simulink model "model"  (R2019b)
settings: Solver=VariableStepAuto  StartTime=0.0  StopTime=sim_time  FixedStep=Ts/100  RelTol=1e-3
StopFcn:
  | %figure;plot(true_position.Data(:,1),true_position.Data(:,2))
  | 
  | figure;hold on;
  | plot(ref_pos.Data(:,1),ref_pos.Data(:,2));
  | plot(ref_pos_noLA.Data(:,1),ref_pos_noLA.Data(:,2));
  | plot(meas_pos.Data(:,1),meas_pos.Data(:,2));
  | title('Position');
  | xlabel('x (m)');
  | ylabel('y (m)');
  | legend('Reference Position','Reference Position without Look-Ahead','Measured Position');
values from neighbouring files (symbols this model uses):
  b = 1.095    [main.m]
  bike_params = [g h b a lambda m]    [main.m]
  complementary = 0.985    [main.m]
  D_balancing = 0.05    [main.m]
  D_heading = 0    [main.m]
  D_lateral = -0.0    (= 0)    [main.m]
  D_steering_position = 0    [main.m]
  g = 9.81    [main.m]
  g1_den = [1]    [main.m]
  g1_num = 3*[1]    [main.m]
  g2_den = [1]    [main.m]
  g2_num = 5*[1]    [main.m]
  heading_control = 1    [main.m]
  I_balancing = 0    [main.m]
  I_heading = 0    [main.m]
  I_lateral = -0.1    [main.m]
  I_steering_position = 30    [main.m]
  IMU_height = 0.45    [main.m]
  initial_roll = deg2rad(0)    [main.m]
  initial_rollrate = deg2rad(0)    [main.m]
  initial_x = 0    [main.m]
  initial_y = 0    [main.m]
  lambda = deg2rad(70)    [main.m]
  lateral_control = 1    [main.m]
  look_ahead = 0    [main.m]
  look_ahead_time = 2.0    (= 2)    [main.m]
  num_tf_steering = [253.4]    [main.m]
  P_balancing = 1    [main.m]
  P_heading = 0.1    [main.m]
  P_lateral = -0.1    [main.m]
  P_steering_position = 30    [main.m]
  path_tracking = 1    [main.m]
  path_x = path_x'    [paths.m]
  path_y = movmean(path_y,200)    [paths.m]
  roll_rate_coef = 0.9    [main.m]
  time_balance = 10    [main.m]
  Ts = 0.01    [main.m]
  v = 4    [main.m]
undefined symbols (not defined in the file or in its folder): A, B, C, cumulative_dist_along_path, curvature, D, den_filt_steeringrate, DiscIntNeverNeededParam, num_filt_steeringrate, Ts_IMU
libraries: simulink_extras x7, simulink x6, dspsigops x3, cstblocks x1
(part 1 of 2)
settings Model: Creator=maximef  LastModifiedBy=maximef
settings DataIOCC: ReturnWorkspaceOutputs=off
settings DebuggingCC: ArithmeticOperatorsInVariantConditions=warning
settings SFSimCC: CustomCodeUndefinedFunction=UseInterfaceOnly

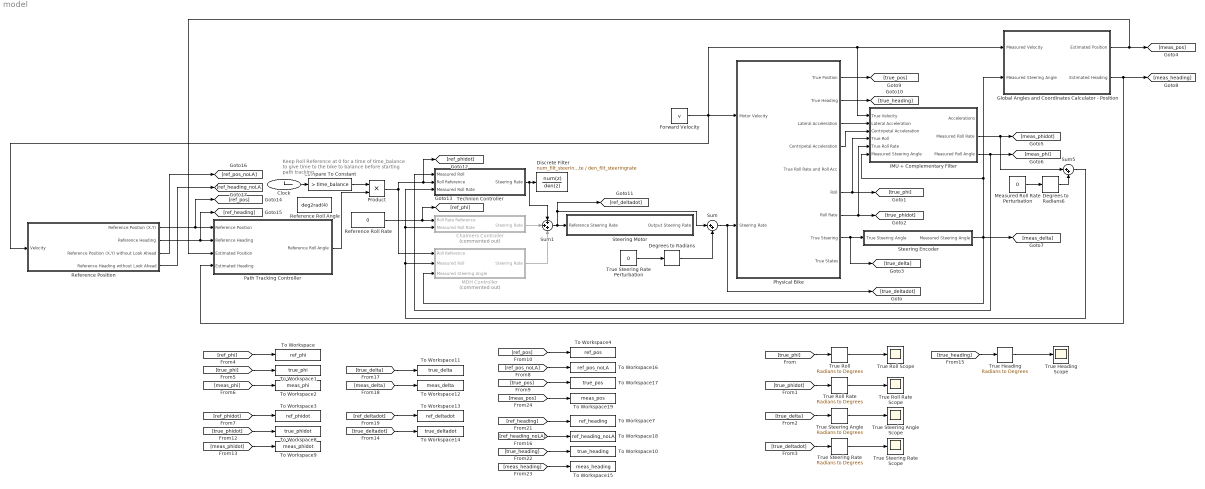
== system model ==
  note: Keep Roll Reference at 0 for a time of time_balance
      | to give time to the bike to balance before starting path tracking
  Chalmers Controller : Subsystem  Commented=on
  Clock : Clock
  Compare To Constant : simulink/Logic and Bit Operations/Compare To Constant  relop=>  const=time_balance  OutDataTypeStr=uint8
  Degrees to Radians : simulink_extras/Transformations/Degrees to Radians
  Degrees to Radians6 : simulink_extras/Transformations/Degrees to Radians
  Discrete Filter : DiscreteFilter  Numerator=num_filt_steeringrate  Denominator=den_filt_steeringrate  SampleTime=Ts
  Forward Velocity : Constant  Value=v
  Global Angles and Coordinates Calculator - Position : Subsystem  TreatAsAtomicUnit=on  SystemSampleTime=Ts
      settings: MinAlgLoopOccurrences=on
  IMU + Complementary Filter : Subsystem  TreatAsAtomicUnit=on
      settings: MinAlgLoopOccurrences=on
  MDH Controller : Subsystem  Commented=on
  Measured Roll Rate Perturbation : Constant  Value=0
  "Path Tracking Controller " : Subsystem  TreatAsAtomicUnit=on
      settings: MinAlgLoopOccurrences=on
  Physical Bike : Subsystem  TreatAsAtomicUnit=on
      settings: MinAlgLoopOccurrences=on
  Product : Product
  Reference Position : Subsystem  TreatAsAtomicUnit=on
      settings: MinAlgLoopOccurrences=on
  Reference Roll Angle : Constant  Value=deg2rad(4)
  Reference Roll Rate : Constant  Value=0
  Steering Encoder : Subsystem  TreatAsAtomicUnit=on  SystemSampleTime=Ts
  Steering Motor : Subsystem  TreatAsAtomicUnit=on
      settings: MinAlgLoopOccurrences=on
  Sum : Sum  Inputs=|++
  Sum1 : Sum  Inputs=+++
  Sum5 : Sum  Inputs=|++
  Technion Controller : Subsystem  TreatAsAtomicUnit=on
      settings: MinAlgLoopOccurrences=on
  To Workspace : ToWorkspace  VariableName=ref_phi  SaveFormat=Timeseries  SampleTime=-1
  To Workspace1 : ToWorkspace  VariableName=true_phi  SaveFormat=Timeseries  SampleTime=-1
  To Workspace10 : ToWorkspace  VariableName=true_heading  SaveFormat=Timeseries  SampleTime=-1
  To Workspace11 : ToWorkspace  VariableName=true_delta  SaveFormat=Timeseries  SampleTime=-1
  To Workspace12 : ToWorkspace  VariableName=meas_delta  SaveFormat=Timeseries  SampleTime=-1
  To Workspace13 : ToWorkspace  VariableName=ref_deltadot  SaveFormat=Timeseries  SampleTime=-1
  To Workspace14 : ToWorkspace  VariableName=true_deltadot  SaveFormat=Timeseries  SampleTime=-1
  To Workspace15 : ToWorkspace  VariableName=meas_heading  SaveFormat=Timeseries  SampleTime=-1
  To Workspace16 : ToWorkspace  VariableName=ref_pos_noLA  SaveFormat=Timeseries  SampleTime=-1
  To Workspace17 : ToWorkspace  VariableName=true_pos  SaveFormat=Timeseries  SampleTime=-1
  To Workspace18 : ToWorkspace  VariableName=ref_heading_noLA  SaveFormat=Timeseries  SampleTime=-1
  To Workspace19 : ToWorkspace  VariableName=meas_pos  SaveFormat=Timeseries  SampleTime=-1
  To Workspace2 : ToWorkspace  VariableName=meas_phi  SaveFormat=Timeseries  SampleTime=-1
  To Workspace3 : ToWorkspace  VariableName=ref_phidot  SaveFormat=Timeseries  SampleTime=-1
  To Workspace4 : ToWorkspace  VariableName=ref_pos  SaveFormat=Timeseries  SampleTime=-1
  To Workspace7 : ToWorkspace  VariableName=ref_heading  SaveFormat=Timeseries  SampleTime=-1
  To Workspace8 : ToWorkspace  VariableName=true_phidot  SaveFormat=Timeseries  SampleTime=-1
  To Workspace9 : ToWorkspace  VariableName=meas_phidot  SaveFormat=Timeseries  SampleTime=-1
  True Heading : simulink_extras/Transformations/Radians to Degrees
  True Heading Scope : Scope
  True Roll : simulink_extras/Transformations/Radians to Degrees
  True Roll Rate : simulink_extras/Transformations/Radians to Degrees
  True Roll Rate Scope : Scope
  True Roll Scope : Scope
  True Steering Angle : simulink_extras/Transformations/Radians to Degrees
  True Steering Angle Scope : Scope
  True Steering Rate : simulink_extras/Transformations/Radians to Degrees
  True Steering Rate Perturbation : Constant  Value=0
  True Steering Rate Scope : Scope
  wires:
  Measured Roll Rate Perturbation/1 -> Degrees to Radians6/1
  Physical Bike/6(Roll) -> [true_phi], IMU + Complementary Filter/4(True Roll)
  Sum/1 -> [true_deltadot], Physical Bike/2(Steering Rate)
  True Steering Rate Perturbation/1 -> Degrees to Radians/1
  Degrees to Radians/1 -> Sum/2
  Degrees to Radians6/1 -> Sum5/2
  Physical Bike/8(True Steering) -> [true_delta], Steering Encoder/1(True Steering Angle)
  Physical Bike/7(Roll Rate) -> [true_phidot], IMU + Complementary Filter/5(True Roll Rate)
  Sum5/1 -> MDH Controller/2(Measured Roll), Chalmers Controller/2(Measured Roll Rate), Technion Controller/3(Measured Roll Rate)
  Sum1/1 -> [ref_deltadot], Sum/1, Steering Motor/1(Reference Steering Rate)
  Steering Encoder/1(Measured Steering Angle) -> [meas_delta], MDH Controller/3(Measured Steering Angle), Global Angles and Coordinates Calculator - Position/2(Measured Steering Angle), IMU + Complementary Filter/6(Measured Steering Angle)
  Reference Position/2(Reference Heading) -> "Path Tracking Controller "/2(Reference Heading), [ref_heading]
  Forward Velocity/1 -> Reference Position/1(Velocity), IMU + Complementary Filter/1(True Velocity), Global Angles and Coordinates Calculator - Position/1(Measured Velocity), Physical Bike/1(Motor Velocity)
  Reference Position/1(Reference Position (X,Y)) -> "Path Tracking Controller "/1(Reference Position), [ref_pos]
  Physical Bike/3(Lateral Acceleration) -> IMU + Complementary Filter/2(Lateral Acceleration)
  Physical Bike/4(Centripetal Acceleration) -> IMU + Complementary Filter/3(Centripetal Acceleration)
  Global Angles and Coordinates Calculator - Position/1(Estimated Position) -> "Path Tracking Controller "/3(Estimated Position), [meas_pos]
  Global Angles and Coordinates Calculator - Position/2(Estimated Heading) -> "Path Tracking Controller "/4(Estimated Heading), [meas_heading]
  IMU + Complementary Filter/2(Measured Roll Rate) -> [meas_phidot], Sum5/1
  IMU + Complementary Filter/3(Measured Roll Angle) -> Technion Controller/1(Measured Roll), [meas_phi]
  Product/1 -> MDH Controller/1(Roll Reference), [ref_phidot], Technion Controller/2(Roll Reference)
  Reference Roll Rate/1 -> [ref_phi], Chalmers Controller/1(Roll Rate Reference)
  True Roll/1 -> True Roll Scope/1
  True Roll Rate/1 -> True Roll Rate Scope/1
  True Steering Angle/1 -> True Steering Angle Scope/1
  Physical Bike/1(True Position) -> [true_pos]
  Physical Bike/2(True Heading) -> [true_heading]
  [true_phi] -> True Roll/1
  [true_phidot] -> True Roll Rate/1
  [true_delta] -> True Steering Angle/1
  [true_deltadot] -> True Steering Rate/1
  True Steering Rate/1 -> True Steering Rate Scope/1
  [true_phi] -> To Workspace1/1
  [ref_phi] -> To Workspace/1
  [meas_phi] -> To Workspace2/1
  [ref_phidot] -> To Workspace3/1
  [meas_phidot] -> To Workspace9/1
  [true_phidot] -> To Workspace8/1
  [true_deltadot] -> To Workspace14/1
  [ref_deltadot] -> To Workspace13/1
  [meas_delta] -> To Workspace12/1
  [true_delta] -> To Workspace11/1
  [ref_heading] -> To Workspace7/1
  [ref_pos] -> To Workspace4/1
  [true_heading] -> True Heading/1
  True Heading/1 -> True Heading Scope/1
  Chalmers Controller/1(Steering Rate) -> Sum1/2
  MDH Controller/1(Steering Rate) -> Sum1/3
  Technion Controller/1(Steering Rate) -> Sum1/1, Discrete Filter/1
  Reference Position/3(Reference Position (X,Y) without Look Ahead) -> [ref_pos_noLA]
  Reference Position/4(Reference Heading without Look Ahead) -> [ref_heading_noLA]
  [meas_heading] -> To Workspace15/1
  [ref_heading_noLA] -> To Workspace18/1
  [true_heading] -> To Workspace10/1
  [true_pos] -> To Workspace17/1
  [ref_pos_noLA] -> To Workspace16/1
  [meas_pos] -> To Workspace19/1
  Clock/1 -> Compare To Constant/1
  "Path Tracking Controller "/1(Reference Roll Angle) -> Product/2
  Compare To Constant/1 -> Product/1

== system model/Chalmers Controller ==
  Roll Rate Reference : Inport
  Measured Roll Rate : Inport  Port=2
  Balance controller : simulink/Continuous/PID Controller  Controller=PID  Form=Parallel  TimeDomain=Discrete-time  SampleTime=Ts  IntegratorMethod=Forward Euler  FilterMethod=Forward Euler  ControllerParametersSource=internal  P=P_balancing  I=I_balancing  D=D_balancing  UseFilter=off  N=5  TunerSelectOption=Transfer Function Based (PID Tuner App)  InitialConditionSource=internal  InitialConditionForIntegrator=0  InitialConditionForFilter=0  DifferentiatorICPrevScaledInput=0  ExternalReset=none  TrackingMode=off  Kt=1  LimitOutput=off  UpperSaturationLimit=inf  LowerSaturationLimit=-inf  LinearizeAsGain=on  AntiWindupMode=none  Kb=1  POutMin=[]  POutMax=[]  IOutMin=[]  IOutMax=[]  DOutMin=[]  DOutMax=[]  NOutMin=[]  NOutMax=[]  SumOutMin=[]  SumOutMax=[]  SaturationOutMin=[]  SaturationOutMax=[]  PParamMin=[]  PParamMax=[]  IParamMin=[]  IParamMax=[]  DParamMin=[]  DParamMax=[]  NParamMin=[]  NParamMax=[]  KbParamMin=[]  KbParamMax=[]  KtParamMin=[]  KtParamMax=[]  KbOutMin=[]  KbOutMax=[]  KtOutMin=[]  KtOutMax=[]  IntegratorOutMin=[]  IntegratorOutMax=[]  FilterOutMin=[]  FilterOutMax=[]  SumI1OutMin=[]  SumI1OutMax=[]  SumI2OutMin=[]  SumI2OutMax=[]  SumI3OutMin=[]  SumI3OutMax=[]  SumI4OutMin=[]  SumI4OutMax=[]  SumDOutMin=[]  SumDOutMax=[]  DifferentiatorOutMin=[]  DifferentiatorOutMax=[]  FilterDiffOutCoefMin=[]  FilterDiffOutCoefMax=[]  ReciprocalOutMin=[]  ReciprocalOutMax=[]  SumDenOutMin=[]  SumDenOutMax=[]  SumNumOutMin=[]  SumNumOutMax=[]  DivideOutMin=[]  DivideOutMax=[]  IntegratorContinuousStateAttributes=''  IntegratorStateMustResolveToSignalObject=off  IntegratorRTWStateStorageClass=Auto  FilterContinuousStateAttributes=''  FilterStateMustResolveToSignalObject=off  FilterRTWStateStorageClass=Auto  ParallelPVariant=InternalParameters  IdealPVariant=Disabled  IVariant=InternalParameters  DVariant=InternalParameters  IntegratorVariant=Discrete  SatVariant=Disabled  AWVariant=Passthrough  PCopyVariant=Disabled  TRVariant=Disabled  FdbkBlocksVariant=Forward  IdealPFdbkVariant=Disabled  SatFdbkVariant=Disabled  DerivativeFilterVariant=Differentiator  NVariant=Passthrough  NCopyVariant=Disabled_SignalSpec  FilterICVariant=InternalICsDifferentiator  IntegratorICVariant=InternalICs  ExternalResetVariant=Disabled  TRSumVariant=Passthrough  SumFdbkVariant=Disabled  SumVariant=Sum_PID
  Sum1 : Sum  Inputs=|+-
  Steering Rate : Outport
  wires:
  Sum1/1 -> Balance controller/1
  Balance controller/1 -> Steering Rate/1
  Measured Roll Rate/1 -> Sum1/2
  Roll Rate Reference/1 -> Sum1/1

== system model/Global Angles and Coordinates Calculator - Position ==
  Measured Velocity : Inport
  Measured Steering Angle : Inport  Port=2
  Gain1 : Gain  Gain=sin(lambda)
  Measured Bike Angles to Global Angles : Subsystem
  Measured Global Angles to Global Coordinates : Subsystem
  Sum : Sum  Inputs=++|
  Estimated Position : Outport  VectorParamsAs1DForOutWhenUnconnected=off
  Estimated Heading : Outport  Port=2  VectorParamsAs1DForOutWhenUnconnected=off
  wires:
  Measured Bike Angles to Global Angles/1(Psi) -> Sum/2, Measured Global Angles to Global Coordinates/2(Psi)
  Gain1/1 -> Measured Bike Angles to Global Angles/2(Measured Steering Angle)
  Sum/1 -> Estimated Heading/1
  Measured Bike Angles to Global Angles/2(Beta) -> Sum/1, Measured Global Angles to Global Coordinates/3(Beta)
  Measured Global Angles to Global Coordinates/1("Position (X, Y)") -> Estimated Position/1
  Measured Velocity/1 -> Measured Global Angles to Global Coordinates/1(Velocity), Measured Bike Angles to Global Angles/1(Velocity)
  Measured Steering Angle/1 -> Gain1/1

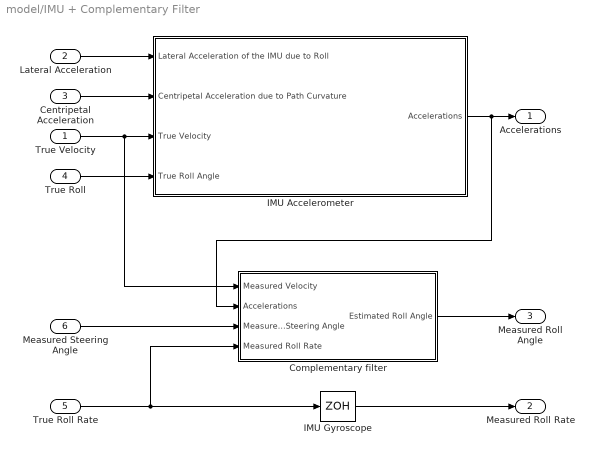
== system model/IMU + Complementary Filter ==
  True Velocity : Inport
  Lateral Acceleration : Inport  Port=2
  Centripetal Acceleration : Inport  Port=3
  True Roll : Inport  Port=4
  True Roll Rate : Inport  Port=5
  Measured Steering Angle : Inport  Port=6
  Complementary filter : Subsystem  SystemSampleTime=Ts_IMU
  IMU Accelerometer : Subsystem
  IMU Gyroscope : ZeroOrderHold  SampleTime=-1
  Accelerations : Outport  VectorParamsAs1DForOutWhenUnconnected=off
  Measured Roll Rate : Outport  Port=2  VectorParamsAs1DForOutWhenUnconnected=off
  Measured Roll Angle : Outport  Port=3  VectorParamsAs1DForOutWhenUnconnected=off
  wires:
  True Velocity/1 -> Complementary filter/1(Measured Velocity), IMU Accelerometer/3(True Velocity)
  Lateral Acceleration/1 -> IMU Accelerometer/1(Lateral Acceleration of the IMU due to Roll)
  Centripetal Acceleration/1 -> IMU Accelerometer/2(Centripetal Acceleration due to Path Curvature)
  True Roll/1 -> IMU Accelerometer/4(True Roll Angle)
  IMU Accelerometer/1(Accelerations) -> Complementary filter/2(Accelerations), Accelerations/1
  IMU Gyroscope/1 -> Measured Roll Rate/1
  True Roll Rate/1 -> Complementary filter/4(Measured Roll Rate), IMU Gyroscope/1
  Complementary filter/1(Estimated Roll Angle) -> Measured Roll Angle/1
  Measured Steering Angle/1 -> Complementary filter/3(Measured Steering Angle)

== system model/MDH Controller ==
  Roll Reference : Inport
  Measured Roll : Inport  Port=2
  Measured Steering Angle : Inport  Port=3
  Balance controller : simulink/Continuous/PID Controller  Controller=PID  Form=Parallel  TimeDomain=Discrete-time  SampleTime=Ts  IntegratorMethod=Forward Euler  FilterMethod=Forward Euler  ControllerParametersSource=internal  P=P_balancing  I=I_balancing  D=D_balancing  UseFilter=off  N=5  TunerSelectOption=Transfer Function Based (PID Tuner App)  InitialConditionSource=internal  InitialConditionForIntegrator=0  InitialConditionForFilter=0  DifferentiatorICPrevScaledInput=0  ExternalReset=none  TrackingMode=off  Kt=1  LimitOutput=off  UpperSaturationLimit=inf  LowerSaturationLimit=-inf  LinearizeAsGain=on  AntiWindupMode=none  Kb=1  POutMin=[]  POutMax=[]  IOutMin=[]  IOutMax=[]  DOutMin=[]  DOutMax=[]  NOutMin=[]  NOutMax=[]  SumOutMin=[]  SumOutMax=[]  SaturationOutMin=[]  SaturationOutMax=[]  PParamMin=[]  PParamMax=[]  IParamMin=[]  IParamMax=[]  DParamMin=[]  DParamMax=[]  NParamMin=[]  NParamMax=[]  KbParamMin=[]  KbParamMax=[]  KtParamMin=[]  KtParamMax=[]  KbOutMin=[]  KbOutMax=[]  KtOutMin=[]  KtOutMax=[]  IntegratorOutMin=[]  IntegratorOutMax=[]  FilterOutMin=[]  FilterOutMax=[]  SumI1OutMin=[]  SumI1OutMax=[]  SumI2OutMin=[]  SumI2OutMax=[]  SumI3OutMin=[]  SumI3OutMax=[]  SumI4OutMin=[]  SumI4OutMax=[]  SumDOutMin=[]  SumDOutMax=[]  DifferentiatorOutMin=[]  DifferentiatorOutMax=[]  FilterDiffOutCoefMin=[]  FilterDiffOutCoefMax=[]  ReciprocalOutMin=[]  ReciprocalOutMax=[]  SumDenOutMin=[]  SumDenOutMax=[]  SumNumOutMin=[]  SumNumOutMax=[]  DivideOutMin=[]  DivideOutMax=[]  IntegratorContinuousStateAttributes=''  IntegratorStateMustResolveToSignalObject=off  IntegratorRTWStateStorageClass=Auto  FilterContinuousStateAttributes=''  FilterStateMustResolveToSignalObject=off  FilterRTWStateStorageClass=Auto  ParallelPVariant=InternalParameters  IdealPVariant=Disabled  IVariant=InternalParameters  DVariant=InternalParameters  IntegratorVariant=Discrete  SatVariant=Disabled  AWVariant=Passthrough  PCopyVariant=Disabled  TRVariant=Disabled  FdbkBlocksVariant=Forward  IdealPFdbkVariant=Disabled  SatFdbkVariant=Disabled  DerivativeFilterVariant=Differentiator  NVariant=Passthrough  NCopyVariant=Disabled_SignalSpec  FilterICVariant=InternalICsDifferentiator  IntegratorICVariant=InternalICs  ExternalResetVariant=Disabled  TRSumVariant=Passthrough  SumFdbkVariant=Disabled  SumVariant=Sum_PID
  Steering Controller : simulink/Continuous/PID Controller  Controller=PID  Form=Parallel  TimeDomain=Discrete-time  SampleTime=Ts  IntegratorMethod=Forward Euler  FilterMethod=Forward Euler  ControllerParametersSource=internal  P=P_steering_position  I=I_steering_position  D=D_steering_position  UseFilter=off  N=100  TunerSelectOption=Transfer Function Based (PID Tuner App)  InitialConditionSource=internal  InitialConditionForIntegrator=0  InitialConditionForFilter=0  DifferentiatorICPrevScaledInput=0  ExternalReset=none  TrackingMode=off  Kt=1  LimitOutput=off  UpperSaturationLimit=inf  LowerSaturationLimit=-inf  LinearizeAsGain=on  AntiWindupMode=none  Kb=1  POutMin=[]  POutMax=[]  IOutMin=[]  IOutMax=[]  DOutMin=[]  DOutMax=[]  NOutMin=[]  NOutMax=[]  SumOutMin=[]  SumOutMax=[]  SaturationOutMin=[]  SaturationOutMax=[]  PParamMin=[]  PParamMax=[]  IParamMin=[]  IParamMax=[]  DParamMin=[]  DParamMax=[]  NParamMin=[]  NParamMax=[]  KbParamMin=[]  KbParamMax=[]  KtParamMin=[]  KtParamMax=[]  KbOutMin=[]  KbOutMax=[]  KtOutMin=[]  KtOutMax=[]  IntegratorOutMin=[]  IntegratorOutMax=[]  FilterOutMin=[]  FilterOutMax=[]  SumI1OutMin=[]  SumI1OutMax=[]  SumI2OutMin=[]  SumI2OutMax=[]  SumI3OutMin=[]  SumI3OutMax=[]  SumI4OutMin=[]  SumI4OutMax=[]  SumDOutMin=[]  SumDOutMax=[]  DifferentiatorOutMin=[]  DifferentiatorOutMax=[]  FilterDiffOutCoefMin=[]  FilterDiffOutCoefMax=[]  ReciprocalOutMin=[]  ReciprocalOutMax=[]  SumDenOutMin=[]  SumDenOutMax=[]  SumNumOutMin=[]  SumNumOutMax=[]  DivideOutMin=[]  DivideOutMax=[]  IntegratorContinuousStateAttributes=''  IntegratorStateMustResolveToSignalObject=off  IntegratorRTWStateStorageClass=Auto  FilterContinuousStateAttributes=''  FilterStateMustResolveToSignalObject=off  FilterRTWStateStorageClass=Auto  ParallelPVariant=InternalParameters  IdealPVariant=Disabled  IVariant=InternalParameters  DVariant=InternalParameters  IntegratorVariant=Discrete  SatVariant=Disabled  AWVariant=Passthrough  PCopyVariant=Disabled  TRVariant=Disabled  FdbkBlocksVariant=Forward  IdealPFdbkVariant=Disabled  SatFdbkVariant=Disabled  DerivativeFilterVariant=Differentiator  NVariant=Passthrough  NCopyVariant=Disabled_SignalSpec  FilterICVariant=InternalICsDifferentiator  IntegratorICVariant=InternalICs  ExternalResetVariant=Disabled  TRSumVariant=Passthrough  SumFdbkVariant=Disabled  SumVariant=Sum_PID
  Sum1 : Sum  Inputs=|+-
  Sum2 : Sum  Inputs=|+-
  Steering Rate : Outport
  wires:
  Sum2/1 -> Steering Controller/1
  Balance controller/1 -> Sum2/1
  Steering Controller/1 -> Steering Rate/1
  Measured Steering Angle/1 -> Sum2/2
  Measured Roll/1 -> Sum1/2
  Sum1/1 -> Balance controller/1
  Roll Reference/1 -> Sum1/1

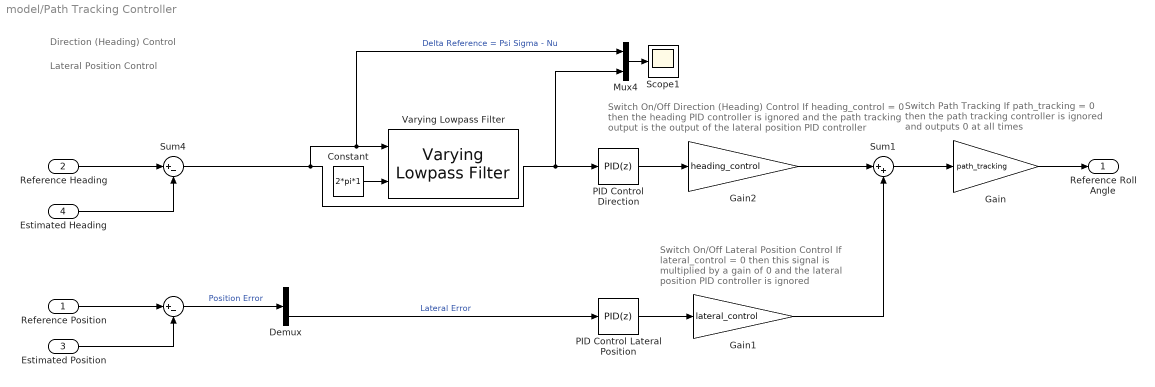
== system model/Path Tracking Controller  ==
  note: Direction (Heading) Control
  note: Lateral Position Control
  note: Switch On/Off Lateral Position Control
      | If lateral_control = 0 then this signal
      | is multiplied by a gain of 0 and the
      | lateral position PID controller is ignored
  note: Switch Path Tracking
      | If path_tracking = 0 then the path tracking controller
      | is ignored and outputs 0 at all times
  note: Switch On/Off Direction (Heading) Control
      | If heading_control = 0 then the heading PID controller is ignored
      | and the path tracking output is the output of the lateral position PID controller
  Reference Position : Inport
  Reference Heading : Inport  Port=2
  Estimated Position : Inport  Port=3
  Estimated Heading : Inport  Port=4
  " " : Sum  Inputs=|+-
  Constant : Constant  Value=2*pi*1
  Demux : Demux  Outputs=2
  Gain : Gain  Gain=path_tracking
  Gain1 : Gain  Gain=lateral_control
  Gain2 : Gain  Gain=heading_control
  Mux4 : Mux  Inputs=2
  PID Control Lateral Position : simulink/Continuous/PID Controller  Controller=PID  Form=Parallel  TimeDomain=Discrete-time  SampleTime=Ts  IntegratorMethod=Forward Euler  FilterMethod=Forward Euler  ControllerParametersSource=internal  P=P_lateral  I=I_lateral  D=D_lateral  UseFilter=on  N=100  TunerSelectOption=Transfer Function Based (PID Tuner App)  InitialConditionSource=internal  InitialConditionForIntegrator=0  InitialConditionForFilter=0  DifferentiatorICPrevScaledInput=0  ExternalReset=none  TrackingMode=off  Kt=1  LimitOutput=off  UpperSaturationLimit=inf  LowerSaturationLimit=-inf  LinearizeAsGain=on  AntiWindupMode=none  Kb=1  POutMin=[]  POutMax=[]  IOutMin=[]  IOutMax=[]  DOutMin=[]  DOutMax=[]  NOutMin=[]  NOutMax=[]  SumOutMin=[]  SumOutMax=[]  SaturationOutMin=[]  SaturationOutMax=[]  PParamMin=[]  PParamMax=[]  IParamMin=[]  IParamMax=[]  DParamMin=[]  DParamMax=[]  NParamMin=[]  NParamMax=[]  KbParamMin=[]  KbParamMax=[]  KtParamMin=[]  KtParamMax=[]  KbOutMin=[]  KbOutMax=[]  KtOutMin=[]  KtOutMax=[]  IntegratorOutMin=[]  IntegratorOutMax=[]  FilterOutMin=[]  FilterOutMax=[]  SumI1OutMin=[]  SumI1OutMax=[]  SumI2OutMin=[]  SumI2OutMax=[]  SumI3OutMin=[]  SumI3OutMax=[]  SumI4OutMin=[]  SumI4OutMax=[]  SumDOutMin=[]  SumDOutMax=[]  DifferentiatorOutMin=[]  DifferentiatorOutMax=[]  FilterDiffOutCoefMin=[]  FilterDiffOutCoefMax=[]  ReciprocalOutMin=[]  ReciprocalOutMax=[]  SumDenOutMin=[]  SumDenOutMax=[]  SumNumOutMin=[]  SumNumOutMax=[]  DivideOutMin=[]  DivideOutMax=[]  IntegratorContinuousStateAttributes=''  IntegratorStateMustResolveToSignalObject=off  IntegratorRTWStateStorageClass=Auto  FilterContinuousStateAttributes=''  FilterStateMustResolveToSignalObject=off  FilterRTWStateStorageClass=Auto  ParallelPVariant=InternalParameters  IdealPVariant=Disabled  IVariant=InternalParameters  DVariant=InternalParameters  IntegratorVariant=Discrete  SatVariant=Disabled  AWVariant=Passthrough  PCopyVariant=Disabled  TRVariant=Disabled  FdbkBlocksVariant=Forward  IdealPFdbkVariant=Disabled  SatFdbkVariant=Disabled  DerivativeFilterVariant=ForwardEulerFilter  NVariant=InternalParameters  NCopyVariant=Disabled  FilterICVariant=InternalICsFilter  IntegratorICVariant=InternalICs  ExternalResetVariant=Disabled  TRSumVariant=Passthrough  SumFdbkVariant=Disabled  SumVariant=Sum_PID
  PID Control Direction : simulink/Continuous/PID Controller  Controller=PID  Form=Parallel  TimeDomain=Discrete-time  SampleTime=Ts  IntegratorMethod=Forward Euler  FilterMethod=Forward Euler  ControllerParametersSource=internal  P=P_heading  I=I_heading  D=D_heading  UseFilter=off  N=100  TunerSelectOption=Transfer Function Based (PID Tuner App)  InitialConditionSource=internal  InitialConditionForIntegrator=0  InitialConditionForFilter=0  DifferentiatorICPrevScaledInput=0  ExternalReset=none  TrackingMode=off  Kt=1  LimitOutput=off  UpperSaturationLimit=inf  LowerSaturationLimit=-inf  LinearizeAsGain=on  AntiWindupMode=none  Kb=1  POutMin=[]  POutMax=[]  IOutMin=[]  IOutMax=[]  DOutMin=[]  DOutMax=[]  NOutMin=[]  NOutMax=[]  SumOutMin=[]  SumOutMax=[]  SaturationOutMin=[]  SaturationOutMax=[]  PParamMin=[]  PParamMax=[]  IParamMin=[]  IParamMax=[]  DParamMin=[]  DParamMax=[]  NParamMin=[]  NParamMax=[]  KbParamMin=[]  KbParamMax=[]  KtParamMin=[]  KtParamMax=[]  KbOutMin=[]  KbOutMax=[]  KtOutMin=[]  KtOutMax=[]  IntegratorOutMin=[]  IntegratorOutMax=[]  FilterOutMin=[]  FilterOutMax=[]  SumI1OutMin=[]  SumI1OutMax=[]  SumI2OutMin=[]  SumI2OutMax=[]  SumI3OutMin=[]  SumI3OutMax=[]  SumI4OutMin=[]  SumI4OutMax=[]  SumDOutMin=[]  SumDOutMax=[]  DifferentiatorOutMin=[]  DifferentiatorOutMax=[]  FilterDiffOutCoefMin=[]  FilterDiffOutCoefMax=[]  ReciprocalOutMin=[]  ReciprocalOutMax=[]  SumDenOutMin=[]  SumDenOutMax=[]  SumNumOutMin=[]  SumNumOutMax=[]  DivideOutMin=[]  DivideOutMax=[]  IntegratorContinuousStateAttributes=''  IntegratorStateMustResolveToSignalObject=off  IntegratorRTWStateStorageClass=Auto  FilterContinuousStateAttributes=''  FilterStateMustResolveToSignalObject=off  FilterRTWStateStorageClass=Auto  ParallelPVariant=InternalParameters  IdealPVariant=Disabled  IVariant=InternalParameters  DVariant=InternalParameters  IntegratorVariant=Discrete  SatVariant=Disabled  AWVariant=Passthrough  PCopyVariant=Disabled  TRVariant=Disabled  FdbkBlocksVariant=Forward  IdealPFdbkVariant=Disabled  SatFdbkVariant=Disabled  DerivativeFilterVariant=Differentiator  NVariant=Passthrough  NCopyVariant=Disabled_SignalSpec  FilterICVariant=InternalICsDifferentiator  IntegratorICVariant=InternalICs  ExternalResetVariant=Disabled  TRSumVariant=Passthrough  SumFdbkVariant=Disabled  SumVariant=Sum_PID
  Scope1 : Scope
  Sum1 : Sum  Inputs=|++
  Sum4 : Sum  Inputs=|+-
  Varying Lowpass Filter : cstblocks/Linear Parameter Varying/Varying Lowpass Filter  N=4
      settings: SourceProductName=Control System Toolbox
  Reference Roll Angle : Outport  VectorParamsAs1DForOutWhenUnconnected=off
  wires:
  Demux/2 -> PID Control Lateral Position/1  "Lateral Error"
  Estimated Position/1 -> " "/2
  " "/1 -> Demux/1  "Position Error"
  Sum4/1 -> Mux4/2, PID Control Direction/1, Mux4/1, Varying Lowpass Filter/1  "Delta Reference = Psi Sigma - Nu"
  Estimated Heading/1 -> Sum4/2
  PID Control Lateral Position/1 -> Gain1/1
  Reference Heading/1 -> Sum4/1
  Reference Position/1 -> " "/1
  Gain2/1 -> Sum1/1
  Sum1/1 -> Gain/1
  Gain/1 -> Reference Roll Angle/1
  PID Control Direction/1 -> Gain2/1
  Gain1/1 -> Sum1/2
  Mux4/1 -> Scope1/1
  Constant/1 -> Varying Lowpass Filter/2

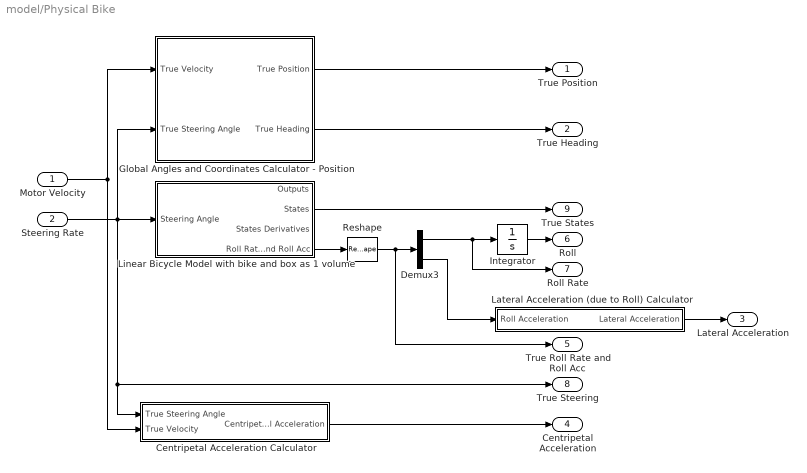
== system model/Physical Bike ==
  Motor Velocity : Inport
  Steering Rate : Inport  Port=2
  Centripetal Acceleration Calculator : Subsystem
  Demux3 : Demux  Outputs=2
  Global Angles and Coordinates Calculator - Position : Subsystem  SystemSampleTime=Ts
  Integrator : Integrator  InitialCondition=initial_roll
  Lateral Acceleration (due to Roll) Calculator : Subsystem
  Linear Bicycle Model with bike and box as 1 volume : Subsystem
  Reshape : Reshape
  True Position : Outport  VectorParamsAs1DForOutWhenUnconnected=off
  True Heading : Outport  Port=2  VectorParamsAs1DForOutWhenUnconnected=off
  Lateral Acceleration : Outport  Port=3  VectorParamsAs1DForOutWhenUnconnected=off
  Centripetal Acceleration : Outport  Port=4  VectorParamsAs1DForOutWhenUnconnected=off
  True Roll Rate and Roll Acc : Outport  Port=5  VectorParamsAs1DForOutWhenUnconnected=off
  Roll : Outport  Port=6  VectorParamsAs1DForOutWhenUnconnected=off
  Roll Rate : Outport  Port=7  VectorParamsAs1DForOutWhenUnconnected=off
  True Steering : Outport  Port=8  VectorParamsAs1DForOutWhenUnconnected=off
  True States : Outport  Port=9  VectorParamsAs1DForOutWhenUnconnected=off
  wires:
  Steering Rate/1 -> Linear Bicycle Model with bike and box as 1 volume/1(Steering Angle), Global Angles and Coordinates Calculator - Position/2(True Steering Angle), True Steering/1, Centripetal Acceleration Calculator/1(True Steering Angle)
  Centripetal Acceleration Calculator/1(Centripetal Acceleration) -> Centripetal Acceleration/1
  Demux3/2 -> Lateral Acceleration (due to Roll) Calculator/1(Roll Acceleration)
  Lateral Acceleration (due to Roll) Calculator/1(Lateral Acceleration) -> Lateral Acceleration/1
  Linear Bicycle Model with bike and box as 1 volume/2(States) -> True States/1
  Demux3/1 -> Integrator/1, Roll Rate/1
  Reshape/1 -> True Roll Rate and Roll Acc/1, Demux3/1
  Linear Bicycle Model with bike and box as 1 volume/4(Roll Rate and Roll Acc) -> Reshape/1
  Motor Velocity/1 -> Centripetal Acceleration Calculator/2(True Velocity), Global Angles and Coordinates Calculator - Position/1(True Velocity)
  Global Angles and Coordinates Calculator - Position/1(True Position) -> True Position/1
  Global Angles and Coordinates Calculator - Position/2(True Heading) -> True Heading/1
  Integrator/1 -> Roll/1

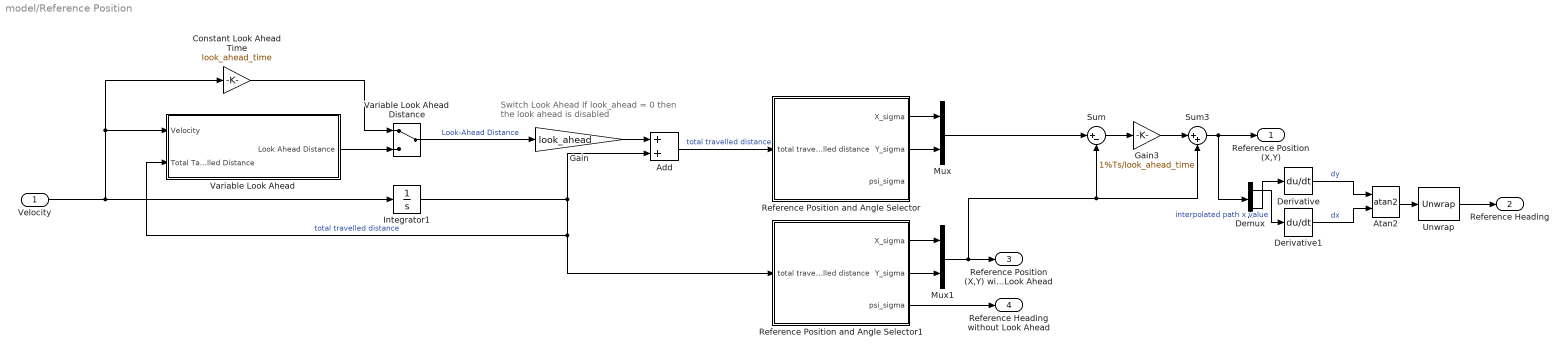
== system model/Reference Position ==
  note: Switch Look Ahead
      | If look_ahead = 0 then the look ahead is disabled
  Velocity : Inport
  Add : Sum
  Atan2 : Trigonometry  Operator=atan2
  Constant Look Ahead Time : Gain  Gain=look_ahead_time
  Demux : Demux  Outputs=2
  Derivative : Derivative
  Derivative1 : Derivative
  Gain : Gain  Gain=look_ahead
  Gain3 : Gain  Gain=1%Ts/look_ahead_time
  Integrator1 : Integrator
  Mux : Mux  Inputs=2
  Mux1 : Mux  Inputs=2
  Reference Position and Angle Selector : Subsystem
  Reference Position and Angle Selector1 : Subsystem
  Sum : Sum  Inputs=|+-
  Sum3 : Sum  Inputs=|++
  Unwrap : dspsigops/Unwrap  tol=pi  InputProcessing=Columns as channels (frame based)  running=off
  Variable Look Ahead Distance : ManualSwitch
  Variable Look Ahead : Subsystem
  Reference Position (X,Y) : Outport  VectorParamsAs1DForOutWhenUnconnected=off
  Reference Heading : Outport  Port=2  VectorParamsAs1DForOutWhenUnconnected=off
  Reference Position (X,Y) without Look Ahead : Outport  Port=3  VectorParamsAs1DForOutWhenUnconnected=off
  Reference Heading without Look Ahead : Outport  Port=4  VectorParamsAs1DForOutWhenUnconnected=off
  wires:
  Velocity/1 -> Integrator1/1, Constant Look Ahead Time/1, Variable Look Ahead/1(Velocity)
  Reference Position and Angle Selector/2(Y_sigma) -> Mux/2
  Add/1 -> Reference Position and Angle Selector/1(total travelled distance)  "total travelled distance"
  Reference Position and Angle Selector/1(X_sigma) -> Mux/1
  Variable Look Ahead Distance/1 -> Gain/1  "Look-Ahead Distance"
  Integrator1/1 -> Add/2, Reference Position and Angle Selector1/1(total travelled distance), Variable Look Ahead/2(Total Tavelled Distance)  "total travelled distance"
  Constant Look Ahead Time/1 -> Variable Look Ahead Distance/1
  Variable Look Ahead/1(Look Ahead Distance) -> Variable Look Ahead Distance/2
  Gain/1 -> Add/1
  Reference Position and Angle Selector1/2(Y_sigma) -> Mux1/2
  Reference Position and Angle Selector1/1(X_sigma) -> Mux1/1
  Mux1/1 -> Sum3/2, Sum/2, Reference Position (X,Y) without Look Ahead/1
  Reference Position and Angle Selector1/3(psi_sigma) -> Reference Heading without Look Ahead/1
  Gain3/1 -> Sum3/1
  Sum/1 -> Gain3/1
  Sum3/1 -> Demux/1, Reference Position (X,Y)/1
  Mux/1 -> Sum/1
  Atan2/1 -> Unwrap/1
  Demux/1 -> Derivative1/1  "interpolated path x value"
  Derivative1/1 -> Atan2/2  "dx"
  Derivative/1 -> Atan2/1  "dy"
  Unwrap/1 -> Reference Heading/1
  Demux/2 -> Derivative/1

== system model/Steering Encoder ==
  True Steering Angle : Inport
  Zero-Order Hold : ZeroOrderHold  SampleTime=Ts
  Measured Steering Angle : Outport  VectorParamsAs1DForOutWhenUnconnected=off
  wires:
  True Steering Angle/1 -> Zero-Order Hold/1
  Zero-Order Hold/1 -> Measured Steering Angle/1

== system model/Steering Motor ==
  Reference Steering Rate : Inport
  Steering motor transfer function Steering Rate reference to Steering Rate : TransferFcn  Numerator=[num_tf_steering]  Denominator=[den_tf_steering(1:end-1)]
  Output Steering Rate : Outport  VectorParamsAs1DForOutWhenUnconnected=off
  wires:
  Steering motor transfer function Steering Rate reference to Steering Rate/1 -> Output Steering Rate/1
  Reference Steering Rate/1 -> Steering motor transfer function Steering Rate reference to Steering Rate/1

== system model/Technion Controller ==
  Measured Roll : Inport
  Roll Reference : Inport  Port=2
  Measured Roll Rate : Inport  Port=3
  G1 : TransferFcn  Numerator=g1_num  Denominator=g1_den
  G2 : TransferFcn  Numerator=g2_num  Denominator=g2_den
  Sum4 : Sum  Inputs=|+-
  Sum6 : Sum  Inputs=|+-
  Steering Rate : Outport
  wires:
  G1/1 -> Sum4/1
  Sum4/1 -> G2/1
  Roll Reference/1 -> Sum6/1
  Sum6/1 -> G1/1
  Measured Roll/1 -> Sum6/2
  G2/1 -> Steering Rate/1
  Measured Roll Rate/1 -> Sum4/2

== system model/Global Angles and Coordinates Calculator - Position/Measured Bike Angles to Global Angles ==
  Velocity : Inport
  Measured Steering Angle : Inport  Port=2
  " Bike Parameters Model " : Constant  Value=bike_params
  Discrete-Time Integrator : DiscreteIntegrator  SampleTime=-1  ICPrevOutput=DiscIntNeverNeededParam  ICPrevScaledInput=DiscIntNeverNeededParam
  Integrator : Integrator  Commented=on
  MATLAB Function : MATLAB Function  TreatAsAtomicUnit=on
  Psi : Outport  VectorParamsAs1DForOutWhenUnconnected=off
  Beta : Outport  Port=2  VectorParamsAs1DForOutWhenUnconnected=off
  wires:
  MATLAB Function/2(beta) -> Beta/1
  MATLAB Function/1(psi_d) -> Discrete-Time Integrator/1
  Discrete-Time Integrator/1 -> Psi/1
  " Bike Parameters Model "/1 -> MATLAB Function/2(parameters_model)
  Measured Steering Angle/1 -> MATLAB Function/3(delta)
  Velocity/1 -> MATLAB Function/1(v)

== system model/Global Angles and Coordinates Calculator - Position/Measured Global Angles to Global Coordinates ==
  Velocity : Inport
  Psi : Inport  Port=2
  Beta : Inport  Port=3
  Discrete-Time Integrator : DiscreteIntegrator  InitialCondition=initial_x  SampleTime=-1  ICPrevOutput=DiscIntNeverNeededParam  ICPrevScaledInput=DiscIntNeverNeededParam
  Discrete-Time Integrator1 : DiscreteIntegrator  InitialCondition=initial_y  SampleTime=-1  ICPrevOutput=DiscIntNeverNeededParam  ICPrevScaledInput=DiscIntNeverNeededParam
  Integrator1 : Integrator  Commented=on  InitialCondition=initial_x
  Integrator2 : Integrator  Commented=on  InitialCondition=initial_y
  MATLAB Function1 : MATLAB Function  TreatAsAtomicUnit=on
  Mux : Mux  Inputs=2
  "Position (X, Y)" : Outport  VectorParamsAs1DForOutWhenUnconnected=off
  wires:
  MATLAB Function1/2(Ydot) -> Discrete-Time Integrator1/1  "Ydot"
  MATLAB Function1/1(Xdot) -> Discrete-Time Integrator/1  "Xdot"
  Psi/1 -> MATLAB Function1/2(psi)
  Beta/1 -> MATLAB Function1/3(beta)
  Velocity/1 -> MATLAB Function1/1(v)
  Discrete-Time Integrator1/1 -> Mux/2
  Discrete-Time Integrator/1 -> Mux/1
  Mux/1 -> "Position (X, Y)"/1

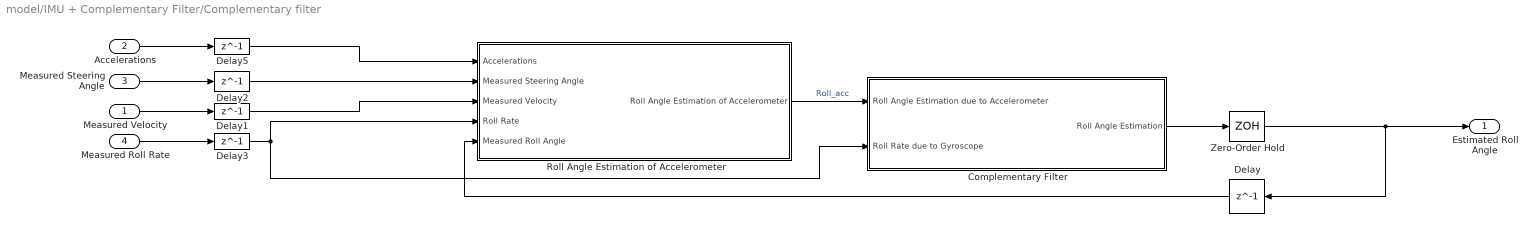
== system model/IMU + Complementary Filter/Complementary filter ==
  Measured Velocity : Inport
  Accelerations : Inport  Port=2
  Measured Steering Angle : Inport  Port=3
  Measured Roll Rate : Inport  Port=4
  Complementary Filter : Subsystem  TreatAsAtomicUnit=on  SystemSampleTime=Ts
  Delay{,1..3,5} (5 alike) : Delay  DelayLength=1
  Roll Angle Estimation of Accelerometer : Subsystem
  Zero-Order Hold : ZeroOrderHold  SampleTime=Ts
  Estimated Roll Angle : Outport  VectorParamsAs1DForOutWhenUnconnected=off
  wires:
  Roll Angle Estimation of Accelerometer/1(Roll Angle Estimation of Accelerometer) -> Complementary Filter/1(Roll Angle Estimation due to Accelerometer)  "Roll_acc"
  Measured Roll Rate/1 -> Delay3/1
  Accelerations/1 -> Delay5/1
  Measured Steering Angle/1 -> Delay2/1
  Measured Velocity/1 -> Delay1/1
  Delay/1 -> Roll Angle Estimation of Accelerometer/5(Measured Roll Angle)
  Delay1/1 -> Roll Angle Estimation of Accelerometer/3(Measured Velocity)
  Delay2/1 -> Roll Angle Estimation of Accelerometer/2(Measured Steering Angle)
  Delay3/1 -> Roll Angle Estimation of Accelerometer/4(Roll Rate), Complementary Filter/2(Roll Rate due to Gyroscope)
  Delay5/1 -> Roll Angle Estimation of Accelerometer/1(Accelerations)
  Complementary Filter/1(Roll Angle Estimation) -> Zero-Order Hold/1
  Zero-Order Hold/1 -> Estimated Roll Angle/1, Delay/1

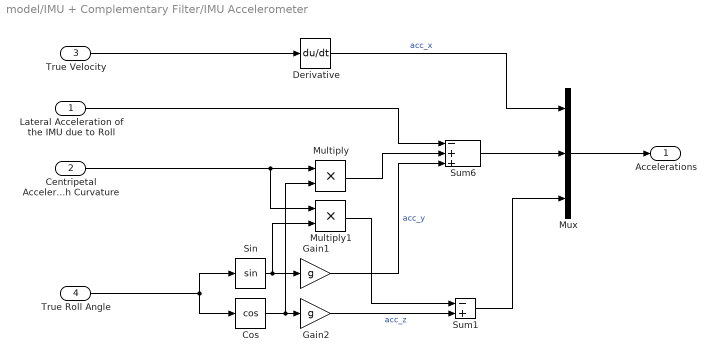
== system model/IMU + Complementary Filter/IMU Accelerometer ==
  Lateral Acceleration of the IMU due to Roll : Inport
  Centripetal Acceleration due to Path Curvature : Inport  Port=2
  True Velocity : Inport  Port=3
  True Roll Angle : Inport  Port=4
  Cos : Trigonometry  Operator=cos
  Derivative : Derivative  CoefficientInTFapproximation=-1
  Gain1 : Gain  Gain=g
  Gain2 : Gain  Gain=g
  Multiply : Product
  Multiply1 : Product
  Mux : Mux  Inputs=3
  Sin : Trigonometry
  Sum1 : Sum  Inputs=-+
  Sum6 : Sum  Inputs=-++
  Accelerations : Outport  VectorParamsAs1DForOutWhenUnconnected=off
  wires:
  Multiply/1 -> Sum6/2
  Gain1/1 -> Sum6/3  "acc_y"
  Sin/1 -> Multiply1/2, Gain1/1
  Derivative/1 -> Mux/1  "acc_x"
  Cos/1 -> Multiply/2, Gain2/1
  Gain2/1 -> Sum1/2  "acc_z"
  True Roll Angle/1 -> Sin/1, Cos/1
  True Velocity/1 -> Derivative/1
  Centripetal Acceleration due to Path Curvature/1 -> Multiply1/1, Multiply/1
  Multiply1/1 -> Sum1/1
  Sum1/1 -> Mux/3
  Mux/1 -> Accelerations/1
  Sum6/1 -> Mux/2
  Lateral Acceleration of the IMU due to Roll/1 -> Sum6/1

== system model/Physical Bike/Centripetal Acceleration Calculator ==
  True Steering Angle : Inport
  True Velocity : Inport  Port=2
  Divide : Product  Inputs=*/
  Gain : Gain  Gain=sin(lambda)
  Multiply : Product
  Square : Math  Operator=square  SaturateOnIntegerOverflow=on
  Tan : Trigonometry  Operator=tan
  b Real Bike : Constant  Value=b
  Centripetal Acceleration : Outport  VectorParamsAs1DForOutWhenUnconnected=off
  wires:
  True Velocity/1 -> Square/1
  Square/1 -> Divide/1
  b Real Bike/1 -> Divide/2
  True Steering Angle/1 -> Gain/1
  Divide/1 -> Multiply/1
  Tan/1 -> Multiply/2
  Multiply/1 -> Centripetal Acceleration/1
  Gain/1 -> Tan/1

== system model/Physical Bike/Global Angles and Coordinates Calculator - Position ==
  note: True Steering
      | Angle
  True Velocity : Inport
  True Steering Angle : Inport  Port=2
  Gain1 : Gain  Gain=sin(lambda)
  Measured Bike Angles to Global Angles : Subsystem
  Measured Global Angles to Global Coordinates : Subsystem
  Sum : Sum  Inputs=++|
  True Position : Outport  VectorParamsAs1DForOutWhenUnconnected=off
  True Heading : Outport  Port=2  VectorParamsAs1DForOutWhenUnconnected=off
  wires:
  Measured Bike Angles to Global Angles/1(Psi) -> Sum/2, Measured Global Angles to Global Coordinates/2(Psi)
  Gain1/1 -> Measured Bike Angles to Global Angles/2(Measured Steering Angle)
  Sum/1 -> True Heading/1
  Measured Bike Angles to Global Angles/2(Beta) -> Sum/1, Measured Global Angles to Global Coordinates/3(Beta)
  Measured Global Angles to Global Coordinates/1("Position (X, Y)") -> True Position/1
  True Velocity/1 -> Measured Global Angles to Global Coordinates/1(Velocity), Measured Bike Angles to Global Angles/1(Velocity)
  True Steering Angle/1 -> Gain1/1

== system model/Physical Bike/Lateral Acceleration (due to Roll) Calculator ==
  Roll Acceleration : Inport
  Constant3 : Constant  Value=IMU_height
  Multiply : Product
  Lateral Acceleration : Outport  VectorParamsAs1DForOutWhenUnconnected=off
  wires:
  Multiply/1 -> Lateral Acceleration/1
  Constant3/1 -> Multiply/1
  Roll Acceleration/1 -> Multiply/2

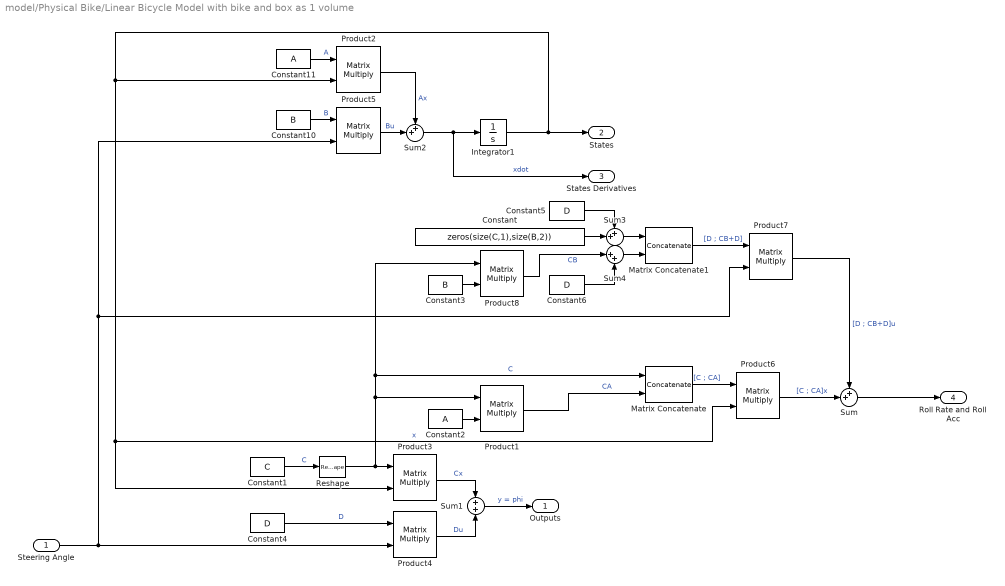
== system model/Physical Bike/Linear Bicycle Model with bike and box as 1 volume ==
  Steering Angle : Inport
  Constant : Constant  Value=zeros(size(C,1),size(B,2))
  Constant1 : Constant  Value=C
  Constant10 : Constant  Value=B
  Constant11 : Constant  Value=A
  Constant2 : Constant  Value=A
  Constant3 : Constant  Value=B
  Constant4 : Constant  Value=D
  Constant5 : Constant  Value=D
  Constant6 : Constant  Value=D
  Integrator1 : Integrator  InitialCondition=[C ; C*A]\[initial_rollrate ; 0]
  Matrix Concatenate : Concatenate  Mode=Multidimensional array
  Matrix Concatenate1 : Concatenate  Mode=Multidimensional array
  Product{1..8} (8 alike) : Product  SCDEnableBlockLinearizationSpecification=on  Multiplication=Matrix(*)
  Reshape : Reshape  OutputDimensionality=Customize  OutputDimensions=[size(C,1),size(C,2)]
  Sum : Sum  Inputs=++|
  Sum1 : Sum
  Sum2 : Sum  Inputs=++|
  Sum3 : Sum  Inputs=++|
  Sum4 : Sum  Inputs=|++
  Outputs : Outport  VectorParamsAs1DForOutWhenUnconnected=off
  States : Outport  Port=2  VectorParamsAs1DForOutWhenUnconnected=off
  States Derivatives : Outport  Port=3  VectorParamsAs1DForOutWhenUnconnected=off
  Roll Rate and Roll Acc : Outport  Port=4  VectorParamsAs1DForOutWhenUnconnected=off
  wires:
  Reshape/1 -> Product3/1, Product8/1, Matrix Concatenate/1, Product1/1  "C"
  Sum/1 -> Roll Rate and Roll Acc/1
  Constant1/1 -> Reshape/1  "C"
  Matrix Concatenate/1 -> Product6/1  "[C ; CA]"
  Product5/1 -> Sum2/2  "Bu"
  Matrix Concatenate1/1 -> Product7/1  "[D ; CB+D]"
  Constant11/1 -> Product2/1  "A"
  Constant3/1 -> Product8/2
  Product6/1 -> Sum/2  "[C ; CA]x"
  Sum2/1 -> Integrator1/1, States Derivatives/1  "xdot"
  Product2/1 -> Sum2/1  "Ax"
  Product1/1 -> Matrix Concatenate/2  "CA"
  Product8/1 -> Sum4/1  "CB"
  Integrator1/1 -> Product2/2, Product6/2, Product3/2, States/1  "x"
  Sum1/1 -> Outputs/1  "y = phi"
  Constant2/1 -> Product1/2
  Product7/1 -> Sum/1  "[D ; CB+D]u"
  Constant10/1 -> Product5/1  "B"
  Steering Angle/1 -> Product4/2, Product5/2, Product7/2
  Product4/1 -> Sum1/2  "Du"
  Product3/1 -> Sum1/1  "Cx"
  Constant4/1 -> Product4/1  "D"
  Sum3/1 -> Matrix Concatenate1/1
  Constant/1 -> Sum3/2
  Constant5/1 -> Sum3/1
  Sum4/1 -> Matrix Concatenate1/2
  Constant6/1 -> Sum4/2

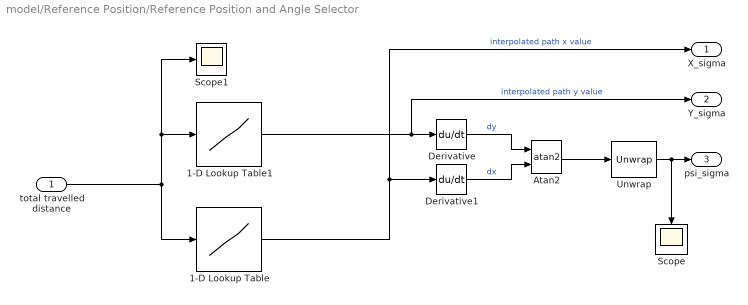
== system model/Reference Position/Reference Position and Angle Selector ==
  total travelled distance : Inport
  1-D Lookup Table : Lookup_n-D  NumberOfTableDimensions=1  BreakpointsForDimension1=cumulative_dist_along_path  Table=path_x  ExtrapMethod=Clip  DiagnosticForOutOfRangeInput=Error  InternalRulePriority=Speed  RndMeth=Simplest  InputSameDT=on
  1-D Lookup Table1 : Lookup_n-D  NumberOfTableDimensions=1  BreakpointsForDimension1=cumulative_dist_along_path  Table=path_y  ExtrapMethod=Clip  DiagnosticForOutOfRangeInput=Error  InternalRulePriority=Speed  RndMeth=Simplest  InputSameDT=on
  Atan2 : Trigonometry  Operator=atan2
  Derivative : Derivative
  Derivative1 : Derivative
  Scope : Scope
  Scope1 : Scope
  Unwrap : dspsigops/Unwrap  tol=pi  InputProcessing=Columns as channels (frame based)  running=off
  X_sigma : Outport  VectorParamsAs1DForOutWhenUnconnected=off
  Y_sigma : Outport  Port=2  VectorParamsAs1DForOutWhenUnconnected=off
  psi_sigma : Outport  Port=3  VectorParamsAs1DForOutWhenUnconnected=off
  wires:
  total travelled distance/1 -> Scope1/1, 1-D Lookup Table1/1, 1-D Lookup Table/1
  Unwrap/1 -> Scope/1, psi_sigma/1
  1-D Lookup Table/1 -> X_sigma/1, Derivative1/1  "interpolated path x value"
  Derivative1/1 -> Atan2/2  "dx"
  Derivative/1 -> Atan2/1  "dy"
  Atan2/1 -> Unwrap/1
  1-D Lookup Table1/1 -> Y_sigma/1, Derivative/1  "interpolated path y value"

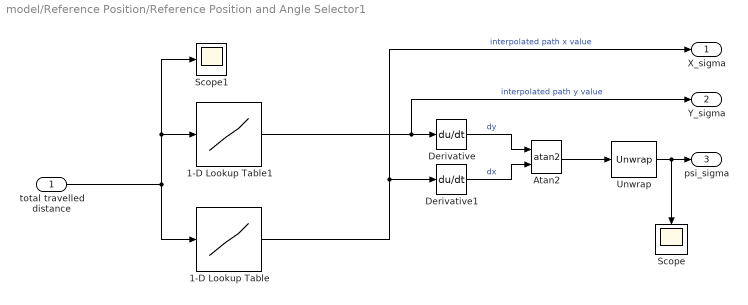
== system model/Reference Position/Reference Position and Angle Selector1 ==
  total travelled distance : Inport
  1-D Lookup Table : Lookup_n-D  NumberOfTableDimensions=1  BreakpointsForDimension1=cumulative_dist_along_path  Table=path_x  ExtrapMethod=Clip  DiagnosticForOutOfRangeInput=Error  InternalRulePriority=Speed  RndMeth=Simplest  InputSameDT=on
  1-D Lookup Table1 : Lookup_n-D  NumberOfTableDimensions=1  BreakpointsForDimension1=cumulative_dist_along_path  Table=path_y  ExtrapMethod=Clip  DiagnosticForOutOfRangeInput=Error  InternalRulePriority=Speed  RndMeth=Simplest  InputSameDT=on
  Atan2 : Trigonometry  Operator=atan2
  Derivative : Derivative
  Derivative1 : Derivative
  Scope : Scope
  Scope1 : Scope
  Unwrap : dspsigops/Unwrap  tol=pi  InputProcessing=Columns as channels (frame based)  running=off
  X_sigma : Outport  VectorParamsAs1DForOutWhenUnconnected=off
  Y_sigma : Outport  Port=2  VectorParamsAs1DForOutWhenUnconnected=off
  psi_sigma : Outport  Port=3  VectorParamsAs1DForOutWhenUnconnected=off
  wires:
  total travelled distance/1 -> Scope1/1, 1-D Lookup Table1/1, 1-D Lookup Table/1
  Unwrap/1 -> Scope/1, psi_sigma/1
  1-D Lookup Table/1 -> X_sigma/1, Derivative1/1  "interpolated path x value"
  Derivative1/1 -> Atan2/2  "dx"
  Derivative/1 -> Atan2/1  "dy"
  Atan2/1 -> Unwrap/1
  1-D Lookup Table1/1 -> Y_sigma/1, Derivative/1  "interpolated path y value"

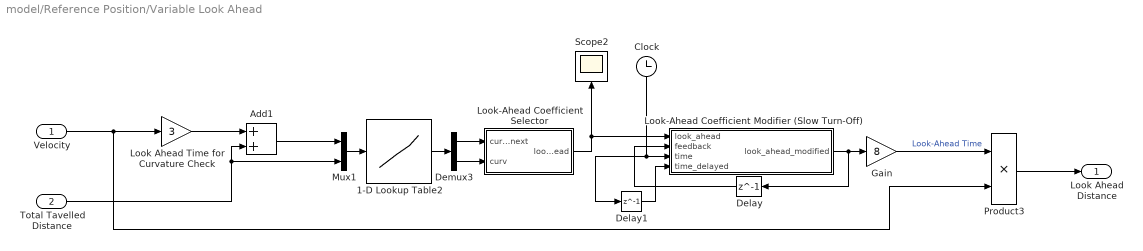
== system model/Reference Position/Variable Look Ahead ==
  Velocity : Inport
  Total Tavelled Distance : Inport  Port=2
  1-D Lookup Table2 : Lookup_n-D  NumberOfTableDimensions=1  BreakpointsForDimension1=cumulative_dist_along_path  Table=curvature  ExtrapMethod=Clip  DiagnosticForOutOfRangeInput=Error  InternalRulePriority=Speed  RndMeth=Simplest  InputSameDT=on
  Add1 : Sum
  Clock : Clock
  Delay : Delay  DelayLength=1
  Delay1 : Delay  DelayLength=1
  Demux3 : Demux  Outputs=2
  Gain : Gain  Gain=8
  Look Ahead Time for Curvature Check : Gain  Gain=3
  Look-Ahead Coefficient Selector : MATLAB Function  TreatAsAtomicUnit=on
  "Look-Ahead Coefficient Modifier (Slow Turn-Off) " : MATLAB Function  TreatAsAtomicUnit=on
  Mux1 : Mux  Inputs=2
  Product3 : Product
  Scope2 : Scope
  Look Ahead Distance : Outport  VectorParamsAs1DForOutWhenUnconnected=off
  wires:
  Look Ahead Time for Curvature Check/1 -> Add1/1
  Delay/1 -> "Look-Ahead Coefficient Modifier (Slow Turn-Off) "/2(feedback)
  "Look-Ahead Coefficient Modifier (Slow Turn-Off) "/1(look_ahead_modified) -> Delay/1, Gain/1
  Demux3/1 -> Look-Ahead Coefficient Selector/1(curv_next)
  Look-Ahead Coefficient Selector/1(look_ahead) -> "Look-Ahead Coefficient Modifier (Slow Turn-Off) "/1(look_ahead), Scope2/1
  Clock/1 -> "Look-Ahead Coefficient Modifier (Slow Turn-Off) "/3(time), Delay1/1
  Delay1/1 -> "Look-Ahead Coefficient Modifier (Slow Turn-Off) "/4(time_delayed)
  1-D Lookup Table2/1 -> Demux3/1
  Total Tavelled Distance/1 -> Mux1/2, Add1/2
  Demux3/2 -> Look-Ahead Coefficient Selector/2(curv)
  Gain/1 -> Product3/1  "Look-Ahead Time"
  Add1/1 -> Mux1/1
  Mux1/1 -> 1-D Lookup Table2/1
  Velocity/1 -> Product3/2, Look Ahead Time for Curvature Check/1
  Product3/1 -> Look Ahead Distance/1

== system model/IMU + Complementary Filter/Complementary filter/Complementary Filter ==
  Roll Angle Estimation due to Accelerometer : Inport
  Roll Rate due to Gyroscope : Inport  Port=2
  Delay : Delay  DelayLength=1  InitialCondition=initial_roll
  Gain2 : Gain  Gain=complementary
  Gain3 : Gain  Gain=1-complementary
  Gain4 : Gain  Gain=Ts
  Sum3 : Sum  Inputs=|++
  Sum4 : Sum  Inputs=++|
  Roll Angle Estimation : Outport  VectorParamsAs1DForOutWhenUnconnected=off
  wires:
  Roll Angle Estimation due to Accelerometer/1 -> Gain3/1  "Roll_acc"
  Sum3/1 -> Gain2/1
  Roll Rate due to Gyroscope/1 -> Gain4/1
  Delay/1 -> Sum3/2
  Gain4/1 -> Sum3/1
  Gain2/1 -> Sum4/2
  Gain3/1 -> Sum4/1
  Sum4/1 -> Delay/1, Roll Angle Estimation/1

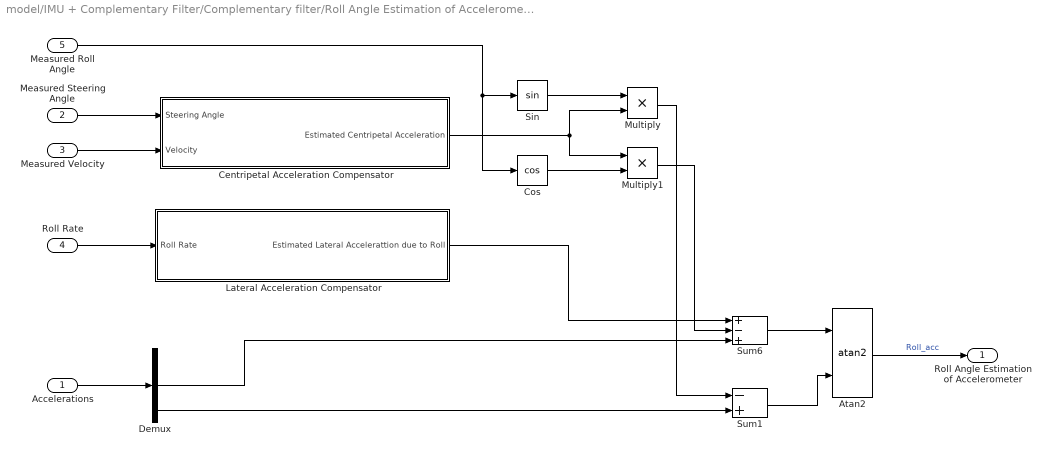
== system model/IMU + Complementary Filter/Complementary filter/Roll Angle Estimation of Accelerometer ==
  Accelerations : Inport
  Measured Steering Angle : Inport  Port=2
  Measured Velocity : Inport  Port=3
  Roll Rate : Inport  Port=4
  Measured Roll Angle : Inport  Port=5
  Atan2 : Trigonometry  Operator=atan2
  Centripetal Acceleration Compensator : Subsystem
  Cos : Trigonometry  Operator=cos
  Demux : Demux  Outputs=3
  Lateral Acceleration Compensator : Subsystem
  Multiply : Product
  Multiply1 : Product
  Sin : Trigonometry
  Sum1 : Sum  Inputs=-+
  Sum6 : Sum  Inputs=+-+
  Roll Angle Estimation of Accelerometer : Outport  VectorParamsAs1DForOutWhenUnconnected=off
  wires:
  Sum1/1 -> Atan2/2
  Lateral Acceleration Compensator/1(Estimated Lateral Accelerattion due to Roll) -> Sum6/1
  Atan2/1 -> Roll Angle Estimation of Accelerometer/1  "Roll_acc"
  Roll Rate/1 -> Lateral Acceleration Compensator/1(Roll Rate)
  Accelerations/1 -> Demux/1
  Measured Velocity/1 -> Centripetal Acceleration Compensator/2(Velocity)
  Centripetal Acceleration Compensator/1(Estimated Centripetal Acceleration) -> Multiply/2, Multiply1/1
  Measured Roll Angle/1 -> Sin/1, Cos/1
  Cos/1 -> Multiply1/2
  Sin/1 -> Multiply/1
  Multiply1/1 -> Sum6/2
  Demux/3 -> Sum1/2
  Multiply/1 -> Sum1/1
  Sum6/1 -> Atan2/1
  Demux/2 -> Sum6/3
  Measured Steering Angle/1 -> Centripetal Acceleration Compensator/1(Steering Angle)

== system model/Physical Bike/Global Angles and Coordinates Calculator - Position/Measured Bike Angles to Global Angles ==
  Velocity : Inport
  Measured Steering Angle : Inport  Port=2
  " Bike Parameters Model " : Constant  Value=bike_params
  Integrator : Integrator
  MATLAB Function : MATLAB Function  TreatAsAtomicUnit=on
  Psi : Outport  VectorParamsAs1DForOutWhenUnconnected=off
  Beta : Outport  Port=2  VectorParamsAs1DForOutWhenUnconnected=off
  wires:
  MATLAB Function/2(beta) -> Beta/1
  MATLAB Function/1(psi_d) -> Integrator/1
  Integrator/1 -> Psi/1
  " Bike Parameters Model "/1 -> MATLAB Function/2(bike_params)
  Measured Steering Angle/1 -> MATLAB Function/3(delta)
  Velocity/1 -> MATLAB Function/1(v)
